simulink model "test_pos"  (R2021a)
settings: Solver=FixedStepAuto  StartTime=0.0  StopTime=25  FixedStep=0.001  RelTol=1e-3
settings Model: Creator=User  LastModifiedBy=User

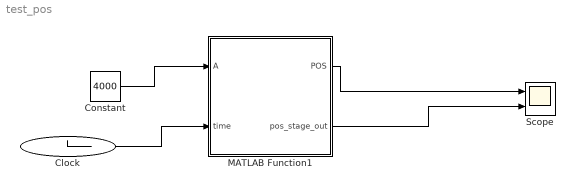
== system test_pos ==
  Clock : Clock
      settings: Decimation=25
  Constant : Constant  Value=4000
  MATLAB Function1 : MATLAB Function  TreatAsAtomicUnit=on
  Scope : Scope  NumInputPorts=2
  wires:
  Constant/1 -> MATLAB Function1/1(A)
  Clock/1 -> MATLAB Function1/2(time)
  MATLAB Function1/1(POS) -> Scope/1
  MATLAB Function1/2(pos_stage_out) -> Scope/2

== matlab function test_pos/MATLAB Function1 ==
  data: A input; POS output; time input; pos_stage_out output
function [POS, pos_stage_out]  = pos_setup(A, time)
persistent pos
if isempty(pos)
    pos = 0;
end

persistent pos_stage
if isempty(pos_stage)
    pos_stage = 0; 
end
    
    
    
pos_count = time *1000;
amplitude = A;
half_amplitude = amplitude *0.5;



    
    
time_0 = 2600;
time_1 = time_0 + 1000;
time_2 = time_1 + amplitude;
time_3 = time_2 + 4000;
time_4 = time_3 + amplitude;
time_5 = time_4 + 3000;
time_6 = time_5 + half_amplitude;
time_7 = time_6 + 2000;
time_8 = time_7 + half_amplitude;
time_9 = time_8 + 3000;

if(pos_count >=time_0 && pos_count <time_1)
    pos_stage = 1;
end

if(pos_count >=time_1 && pos_count <time_2)
    pos_stage = 2;
end
if(pos_count >=time_2 && pos_count <time_3)
    pos_stage = 3;
end
if(pos_count >=time_3 && pos_count <time_4)
    pos_stage = 4;
end
if(pos_count >=time_4 && pos_count <time_5)
    pos_stage = 5;
end

if(pos_count >=time_5 && pos_count <time_6)
    pos_stage = 6;
end
if(pos_count >=time_6 && pos_count <time_7)
    pos_stage = 7;
end
if(pos_count >=time_7 && pos_count <time_8)
    pos_stage = 8;
end
if(pos_count >=time_8 && pos_count <time_9)
    pos_stage = 9;
end

if(pos_count >=time_9)
    pos_stage = 10;
end
            
 
switch pos_stage
        case 1
            pos = 0;
        case 2
            pos = pos - 1;
        case 3
            pos = -1 * amplitude;
        case 4
            pos = pos + 1;
        case 5
            pos = 0;
        case 6
            pos = pos - 1;
        case 7
            pos = -1 * half_amplitude;
        case 8
            pos = pos + 1;
        case 9
            pos = 0;

end


POS = -0.5 *0.025 * pos ;

pos_stage_out = pos_stage *10;
